simulink model "simulate_complexIQTransceiver_AM"  (R2017a)
settings: Solver=VariableStepAuto  StartTime=0.0  StopTime=.1  RelTol=1e-3
InitFcn:
  | fs = 1e4;
  | frameSize = 1000;
libraries: dspsrcs4 x4, dspfdesign x1
settings Model: Creator=prust  LastModifiedBy=prust

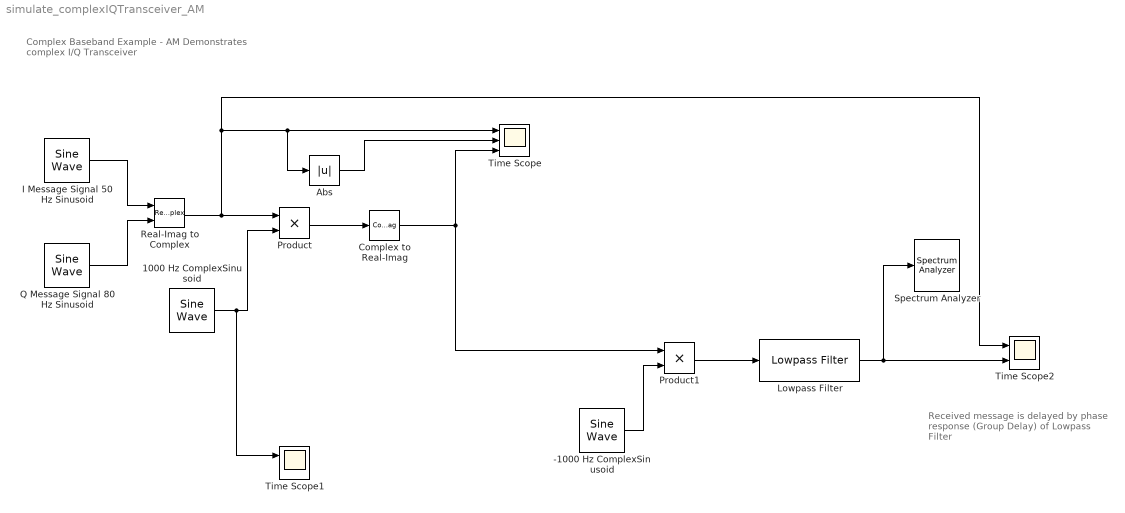
== system simulate_complexIQTransceiver_AM ==
  note: Received message is delayed by phase response (Group Delay) of Lowpass Filter
  note: Complex Baseband Example - AM
      | Demonstrates complex I/Q Transceiver
  -1000 Hz ComplexSinusoid : dspsrcs4/Sine Wave  Amplitude=sqrt(2)  Frequency=-1000  Phase=0  SampleMode=Discrete  OutComplex=Complex  CompMethod=Trigonometric fcn  TableSize=Speed  SampleTime=1/fs  SamplesPerFrame=frameSize  ResetState=Restart at time zero  OutputFrames=off  dataType=double  wordLen=16  udDataType=sfix(16)  fracBitsMode=Best precision  numFracBits=15  OutDataTypeStr=double  LastOutDataTypeStr=double
  1000 Hz ComplexSinusoid : dspsrcs4/Sine Wave  Amplitude=sqrt(2)  Frequency=1000  Phase=0  SampleMode=Discrete  OutComplex=Complex  CompMethod=Trigonometric fcn  TableSize=Speed  SampleTime=1/fs  SamplesPerFrame=frameSize  ResetState=Restart at time zero  OutputFrames=off  dataType=double  wordLen=16  udDataType=sfix(16)  fracBitsMode=Best precision  numFracBits=15  OutDataTypeStr=double  LastOutDataTypeStr=double
  Abs : Abs
  Complex to Real-Imag : ComplexToRealImag  Output=Real
  I Message Signal 50 Hz Sinusoid : dspsrcs4/Sine Wave  Amplitude=1  Frequency=50  Phase=0  SampleMode=Discrete  OutComplex=Real  CompMethod=Trigonometric fcn  TableSize=Speed  SampleTime=1/fs  SamplesPerFrame=frameSize  ResetState=Restart at time zero  OutputFrames=off  dataType=double  wordLen=16  udDataType=sfix(16)  fracBitsMode=Best precision  numFracBits=15  OutDataTypeStr=double  LastOutDataTypeStr=double
  Lowpass Filter : dspfdesign/Lowpass Filter  FilterType=FIR  DesignForMinimumOrder=off  FilterOrder=100  PassbandFrequency=800  StopbandFrequency=1200  PassbandRipple=0.1  StopbandAttenuation=80  InheritSampleRate=off  SampleRate=fs  SimulateUsing=Interpreted execution  roundingMode=Floor  coeffsDataTypeStr=fixdt(1,16)
  Product : Product
  Product1 : Product
  Q Message Signal 80 Hz Sinusoid : dspsrcs4/Sine Wave  Amplitude=1  Frequency=80  Phase=0  SampleMode=Discrete  OutComplex=Real  CompMethod=Trigonometric fcn  TableSize=Speed  SampleTime=1/fs  SamplesPerFrame=frameSize  ResetState=Restart at time zero  OutputFrames=off  dataType=double  wordLen=16  udDataType=sfix(16)  fracBitsMode=Best precision  numFracBits=15  OutDataTypeStr=double  LastOutDataTypeStr=double
  Real-Imag to Complex : RealImagToComplex
  Spectrum Analyzer : SpectrumAnalyzer
  Time Scope : Scope  NumInputPorts=3
  Time Scope1 : Scope  NumInputPorts=2
  Time Scope2 : Scope  NumInputPorts=2
  wires:
  I Message Signal 50 Hz Sinusoid/1 -> Real-Imag to Complex/1
  Q Message Signal 80 Hz Sinusoid/1 -> Real-Imag to Complex/2
  Real-Imag to Complex/1 -> Abs/1, Time Scope/1, Time Scope2/1, Product/1
  1000 Hz ComplexSinusoid/1 -> Time Scope1/1, Product/2
  Product/1 -> Complex to Real-Imag/1
  Abs/1 -> Time Scope/2
  Complex to Real-Imag/1 -> Product1/1, Time Scope/3
  -1000 Hz ComplexSinusoid/1 -> Product1/2
  Product1/1 -> Lowpass Filter/1
  Lowpass Filter/1 -> Time Scope2/2, Spectrum Analyzer/1
